simulink model "discrete_control_angle_from_acc"  (Simulink 7.4)
settings: Solver=ode45  StartTime=0.0  StopTime=30.0  RelTol=1e-3
values from neighbouring files (symbols this model uses):
  phi0 = 0.15    [discrete_control_angle_from_acc_Driver.m]    (also in discrete_control_sfunc_Driver.m)
  r_psi0 = 0.1    [discrete_control_angle_from_acc_Driver.m]    (also in discrete_control_sfunc_Driver.m)
  theta0 = 0.15    [discrete_control_angle_from_acc_Driver.m]    (also in discrete_control_sfunc_Driver.m)
undefined symbols (not defined in the file or in its folder): boom, DiscIntNeverNeededParam, f1, f2, f3, f4, f5, g, I_x, I_y, I_z, Ts
libraries: Copter_Library x5
settings Model: Creator=Robert  LastModifiedBy=roczit00

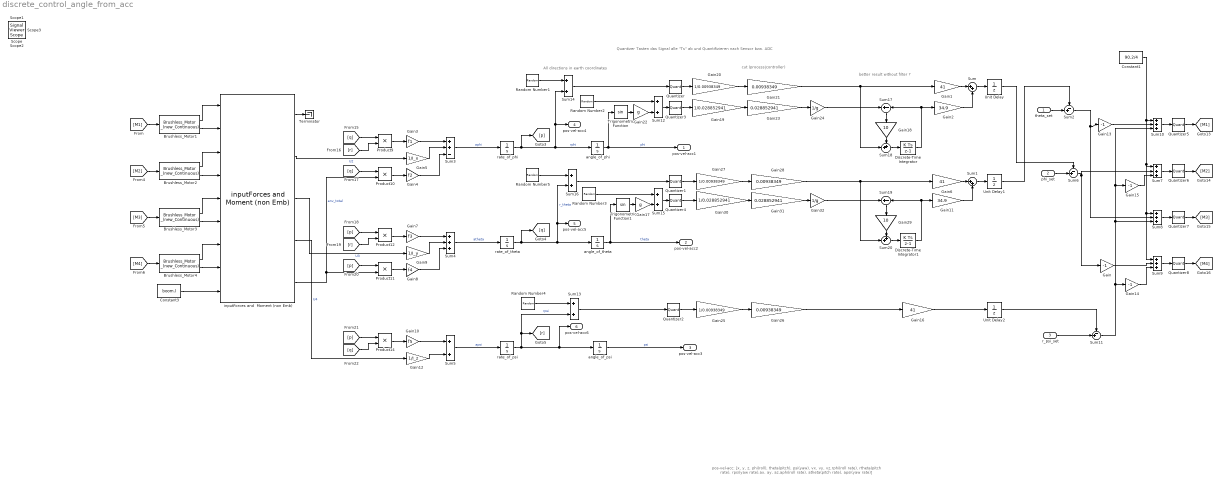
== system discrete_control_angle_from_acc ==
  note: pos-vel-acc: [x, y, z, phi(roll), theta(pitch), psi(yaw), vx, vy, vz,rphi(roll rate), rtheta(pitch rate), rpsi(yaw rate),ax, ay, az,aphi(roll rate), atheta(pitch rate), apsi(yaw rate)]
  note: All directions in earth coordinates
  note: cut (process|controller)
  note: Quantizer Tasten das Signal alle "Ts" ab und Quantifizieren nach Sensor bzw. ADC
  note: better result without filter ?
  theta_set : Inport  OutDataType=fixdt(1, 16)  OutScaling=2^0
  phi_set : Inport  Port=2  OutDataType=fixdt(1, 16)  OutScaling=2^0
  r_psi_set : Inport  Port=3  OutDataType=fixdt(1, 16)  OutScaling=2^0
  Brushless_Motor{1..4} (4 alike) : Copter_Library/Brushless_Motor _(new_Continuous)  SystemSampleTime=-1  M_error=1
  Constant1 : Constant  Value=90.2/4  OutDataType=fixdt(1, 16)  OutScaling=2^0
  Constant3 : Constant  Value=boom.l  OutDataType=fixdt(1, 16)  OutScaling=2^0
  Discrete-Time Integrator : DiscreteIntegrator  InitialCondition=phi0  SampleTime=Ts  OutDataType=fixdt(1, 16)  OutScaling=2^0  ICPrevOutput=DiscIntNeverNeededParam  ICPrevScaledInput=DiscIntNeverNeededParam
  Discrete-Time Integrator1 : DiscreteIntegrator  InitialCondition=theta0  SampleTime=Ts  OutDataType=fixdt(1, 16)  OutScaling=2^0  ICPrevOutput=DiscIntNeverNeededParam  ICPrevScaledInput=DiscIntNeverNeededParam
  Gain{,13..15} (4 alike) : Gain  Gain=-1  ParameterDataType=fixdt(1, 16)  ParameterScaling=2^0  OutDataType=fixdt(1, 16)  OutScaling=2^0
  Gain1 : Gain  Gain=41  ParameterDataType=fixdt(1, 16)  ParameterScaling=2^0  OutDataType=fixdt(1, 16)  OutScaling=2^0
  Gain10 : Gain  Gain=f5  ParameterDataType=fixdt(1, 16)  ParameterScaling=2^0  OutDataType=fixdt(1, 16)  OutScaling=2^0
  Gain11 : Gain  Gain=34.9  ParameterDataType=fixdt(1, 16)  ParameterScaling=2^0  OutDataType=fixdt(1, 16)  OutScaling=2^0
  Gain12 : Gain  Gain=1/I_z  ParameterDataType=fixdt(1, 16)  ParameterScaling=2^0  OutDataType=fixdt(1, 16)  OutScaling=2^0
  Gain16 : Gain  Gain=41  ParameterDataType=fixdt(1, 16)  ParameterScaling=2^0  OutDataType=fixdt(1, 16)  OutScaling=2^0
  Gain17 : Gain  Gain=g  ParameterDataType=fixdt(1, 16)  ParameterScaling=2^0  OutDataType=fixdt(1, 16)  OutScaling=2^0
  Gain18 : Gain  Gain=10  ParameterDataType=fixdt(1, 16)  ParameterScaling=2^0  OutDataType=fixdt(1, 16)  OutScaling=2^0
  Gain19 : Gain  Gain=1/0.028852941  ParameterDataType=fixdt(1, 16)  ParameterScaling=2^0  OutDataType=fixdt(1, 16)  OutScaling=2^0
  Gain2 : Gain  Gain=34.9  ParameterDataType=fixdt(1, 16)  ParameterScaling=2^0  OutDataType=fixdt(1, 16)  OutScaling=2^0
  Gain20 : Gain  Gain=1/0.00938349  ParameterDataType=fixdt(1, 16)  ParameterScaling=2^0  OutDataType=fixdt(1, 16)  OutScaling=2^0
  Gain21 : Gain  Gain=0.00938349  ParameterDataType=fixdt(1, 16)  ParameterScaling=2^0  OutDataType=fixdt(1, 16)  OutScaling=2^0
  Gain22 : Gain  Gain=g  ParameterDataType=fixdt(1, 16)  ParameterScaling=2^0  OutDataType=fixdt(1, 16)  OutScaling=2^0
  Gain23 : Gain  Gain=0.028852941  ParameterDataType=fixdt(1, 16)  ParameterScaling=2^0  OutDataType=fixdt(1, 16)  OutScaling=2^0
  Gain24 : Gain  Gain=1/g  ParameterDataType=fixdt(1, 16)  ParameterScaling=2^0  OutDataType=fixdt(1, 16)  OutScaling=2^0
  Gain25 : Gain  Gain=1/0.00938349  ParameterDataType=fixdt(1, 16)  ParameterScaling=2^0  OutDataType=fixdt(1, 16)  OutScaling=2^0
  Gain26 : Gain  Gain=0.00938349  ParameterDataType=fixdt(1, 16)  ParameterScaling=2^0  OutDataType=fixdt(1, 16)  OutScaling=2^0
  Gain27 : Gain  Gain=1/0.00938349  ParameterDataType=fixdt(1, 16)  ParameterScaling=2^0  OutDataType=fixdt(1, 16)  OutScaling=2^0
  Gain28 : Gain  Gain=0.00938349  ParameterDataType=fixdt(1, 16)  ParameterScaling=2^0  OutDataType=fixdt(1, 16)  OutScaling=2^0
  Gain29 : Gain  Gain=10  ParameterDataType=fixdt(1, 16)  ParameterScaling=2^0  OutDataType=fixdt(1, 16)  OutScaling=2^0
  Gain3 : Gain  Gain=f1  ParameterDataType=fixdt(1, 16)  ParameterScaling=2^0  OutDataType=fixdt(1, 16)  OutScaling=2^0
  Gain30 : Gain  Gain=1/0.028852941  ParameterDataType=fixdt(1, 16)  ParameterScaling=2^0  OutDataType=fixdt(1, 16)  OutScaling=2^0
  Gain31 : Gain  Gain=0.028852941  ParameterDataType=fixdt(1, 16)  ParameterScaling=2^0  OutDataType=fixdt(1, 16)  OutScaling=2^0
  Gain32 : Gain  Gain=1/g  ParameterDataType=fixdt(1, 16)  ParameterScaling=2^0  OutDataType=fixdt(1, 16)  OutScaling=2^0
  Gain4 : Gain  Gain=f2  ParameterDataType=fixdt(1, 16)  ParameterScaling=2^0  OutDataType=fixdt(1, 16)  OutScaling=2^0
  Gain5 : Gain  Gain=1/I_x  ParameterDataType=fixdt(1, 16)  ParameterScaling=2^0  OutDataType=fixdt(1, 16)  OutScaling=2^0
  Gain6 : Gain  Gain=41  ParameterDataType=fixdt(1, 16)  ParameterScaling=2^0  OutDataType=fixdt(1, 16)  OutScaling=2^0
  Gain7 : Gain  Gain=f3  ParameterDataType=fixdt(1, 16)  ParameterScaling=2^0  OutDataType=fixdt(1, 16)  OutScaling=2^0
  Gain8 : Gain  Gain=f4  ParameterDataType=fixdt(1, 16)  ParameterScaling=2^0  OutDataType=fixdt(1, 16)  OutScaling=2^0
  Gain9 : Gain  Gain=1/I_y  ParameterDataType=fixdt(1, 16)  ParameterScaling=2^0  OutDataType=fixdt(1, 16)  OutScaling=2^0
  Product{9..12,14} (5 alike) : Product  OutDataType=fixdt(1, 16)  OutScaling=2^0  RndMeth=Zero
  Quantizer : Quantizer  QuantizationInterval=0.00938349  SampleTime=Ts
  Quantizer1 : Quantizer  QuantizationInterval=0.00938349  SampleTime=Ts
  Quantizer2 : Quantizer  QuantizationInterval=0.00938349  SampleTime=Ts
  Quantizer3 : Quantizer  QuantizationInterval=0.028852941  SampleTime=Ts
  Quantizer4 : Quantizer  QuantizationInterval=0.003  SampleTime=Ts
  Quantizer{5..8} (4 alike) : Quantizer  QuantizationInterval=1  SampleTime=Ts
  Random Number1 : RandomNumber  Variance=3.0462e-8  Seed=45632  SampleTime=0.01
  Random Number2 : RandomNumber  Variance=0.0003  Seed=4564  SampleTime=0.01
  Random Number3 : RandomNumber  Variance=0.0003  Seed=676  SampleTime=Ts
  Random Number4 : RandomNumber  Variance=3.0462e-8  Seed=1634  SampleTime=0.01
  Random Number5 : RandomNumber  Variance=3.0462e-8  Seed=4731  SampleTime=0.01
  Sum : Sum  Inputs=|++  OutDataType=fixdt(1, 16)  OutScaling=2^0
  Sum1 : Sum  Inputs=|++  OutDataType=fixdt(1, 16)  OutScaling=2^0
  Sum{4,7..10} (5 alike) : Sum  Inputs=+++  OutDataType=fixdt(1, 16)  OutScaling=2^0
  Sum11 : Sum  Inputs=-+|  OutDataType=fixdt(1, 16)  OutScaling=2^0
  Sum{5,12..16} (6 alike) : Sum  OutDataType=fixdt(1, 16)  OutScaling=2^0
  Sum17 : Sum  Inputs=+|-  OutDataType=fixdt(1, 16)  OutScaling=2^0
  Sum18 : Sum  Inputs=++|  OutDataType=fixdt(1, 16)  OutScaling=2^0
  Sum19 : Sum  Inputs=+|-  OutDataType=fixdt(1, 16)  OutScaling=2^0
  Sum2 : Sum  Inputs=-+|  OutDataType=fixdt(1, 16)  OutScaling=2^0
  Sum20 : Sum  Inputs=++|  OutDataType=fixdt(1, 16)  OutScaling=2^0
  Sum3 : Sum  Inputs=++-  OutDataType=fixdt(1, 16)  OutScaling=2^0
  Sum6 : Sum  Inputs=-+|  OutDataType=fixdt(1, 16)  OutScaling=2^0
  Terminator : Terminator
  Trigonometric Function : Trigonometry
  Trigonometric Function1 : Trigonometry
  Unit Delay : UnitDelay  SampleTime=Ts
  Unit Delay1 : UnitDelay  SampleTime=Ts
  Unit Delay2 : UnitDelay  SampleTime=Ts
  angle_of_phi : Integrator  InitialCondition=phi0
  angle_of_psi : Integrator
  angle_of_theta : Integrator  InitialCondition=theta0
  inputForces and  Moment (non Emb) : Copter_Library/inputForces and  Moment (non Emb)  SystemSampleTime=-1
  rate_of_phi : Integrator
  rate_of_psi : Integrator  InitialCondition=r_psi0
  rate_of_theta : Integrator
  pos-vel-acc1 : Outport  OutDataType=fixdt(1, 16)  OutScaling=2^0
  pos-vel-acc2 : Outport  Port=2  OutDataType=fixdt(1, 16)  OutScaling=2^0
  pos-vel-acc3 : Outport  Port=3  OutDataType=fixdt(1, 16)  OutScaling=2^0
  pos-vel-acc4 : Outport  Port=4  OutDataType=fixdt(1, 16)  OutScaling=2^0
  pos-vel-acc5 : Outport  Port=5  OutDataType=fixdt(1, 16)  OutScaling=2^0
  pos-vel-acc6 : Outport  Port=6  OutDataType=fixdt(1, 16)  OutScaling=2^0
  Scope : SignalViewerScope  IOType=viewer  ZoomMode=yonly  LegendLocations="235.3333           183            72      20.33333"  RefreshTime=0.035000
      settings: ShowLegends=on
  Scope1 : SignalViewerScope  IOType=viewer  ZoomMode=yonly  LegendLocations="225.3333           183            82      20.33333"  RefreshTime=0.035000
      settings: ShowLegends=on
  Scope2 : SignalViewerScope  IOType=viewer  ZoomMode=yonly  LegendLocations="220.3333           183            74      20.33333"  RefreshTime=0.035000
      settings: ShowLegends=on  SaveName=ScopeData2
  Scope3 : SignalViewerScope  IOType=viewer  ZoomMode=xonly  RefreshTime=0.035000
      settings: ShowLegends=on  SaveName=ScopeData3
  wires:
  Constant3/1 -> inputForces and  Moment (non Emb)/9
  Sum5/1 -> rate_of_psi/1  "apsi"
  inputForces and  Moment (non Emb)/4 -> Gain12/1  "U4"
  Gain12/1 -> Sum5/2
  Gain10/1 -> Sum5/1
  Product14/1 -> Gain10/1
  [q] -> Product14/2
  [p] -> Product14/1
  Sum4/1 -> rate_of_theta/1  "atheta"
  inputForces and  Moment (non Emb)/3 -> Gain9/1  "U3"
  Gain8/1 -> Sum4/3
  Gain9/1 -> Sum4/2
  Product11/1 -> Gain8/1
  [p] -> Product11/1
  Gain7/1 -> Sum4/1
  Product12/1 -> Gain7/1
  [r] -> Product12/2
  [p] -> Product12/1
  Sum3/1 -> rate_of_phi/1  "aphi"
  Gain4/1 -> Sum3/3
  Gain5/1 -> Sum3/2
  inputForces and  Moment (non Emb)/2 -> Gain5/1  "U2"
  Product10/1 -> Gain4/1
  [q] -> Product10/1
  Gain3/1 -> Sum3/1
  Product9/1 -> Gain3/1
  [r] -> Product9/2
  [q] -> Product9/1
  inputForces and  Moment (non Emb)/5 -> Product11/2, Product10/2  "anv_total"
  angle_of_phi/1 -> pos-vel-acc1/1, Trigonometric Function/1  "phi"
  angle_of_theta/1 -> pos-vel-acc2/1, Trigonometric Function1/1  "theta"
  angle_of_psi/1 -> pos-vel-acc3/1  "psi"
  rate_of_phi/1 -> [p], angle_of_phi/1, pos-vel-acc4/1, Sum14/2  "rphi"
  rate_of_theta/1 -> angle_of_theta/1, pos-vel-acc5/1, Sum16/2, [q]  "r_theta"
  rate_of_psi/1 -> angle_of_psi/1, pos-vel-acc6/1, [r], Sum13/2  "rpsi"
  Brushless_Motor1/1 -> inputForces and  Moment (non Emb)/1
  Brushless_Motor1/2 -> inputForces and  Moment (non Emb)/2
  Brushless_Motor2/1 -> inputForces and  Moment (non Emb)/3
  Brushless_Motor2/2 -> inputForces and  Moment (non Emb)/4
  Brushless_Motor3/1 -> inputForces and  Moment (non Emb)/5
  Brushless_Motor3/2 -> inputForces and  Moment (non Emb)/6
  Brushless_Motor4/1 -> inputForces and  Moment (non Emb)/7
  Brushless_Motor4/2 -> inputForces and  Moment (non Emb)/8
  Gain1/1 -> Sum/1
  Gain2/1 -> Sum/2
  Gain6/1 -> Sum1/1
  Gain11/1 -> Sum1/2
  inputForces and  Moment (non Emb)/1 -> Terminator/1
  Sum/1 -> Unit Delay/1
  Sum1/1 -> Unit Delay1/1
  Gain16/1 -> Unit Delay2/1
  Random Number2/1 -> Sum12/1
  Random Number1/1 -> Sum14/1
  Random Number3/1 -> Sum15/1
  Random Number5/1 -> Sum16/1
  Random Number4/1 -> Sum13/1
  Sum14/1 -> Quantizer/1
  Sum16/1 -> Quantizer1/1
  Sum13/1 -> Quantizer2/1
  Sum12/1 -> Quantizer3/1
  Sum15/1 -> Quantizer4/1
  Unit Delay2/1 -> Sum11/1
  Unit Delay1/1 -> Sum2/1
  Unit Delay/1 -> Sum6/1
  [M1] -> Brushless_Motor1/1
  theta_set/1 -> Sum2/2
  Sum2/1 -> Gain13/1, Sum8/2
  phi_set/1 -> Sum6/2
  Sum6/1 -> Gain/1, Sum7/2
  Constant1/1 -> Sum10/1, Sum7/1, Sum8/1, Sum9/1
  Gain13/1 -> Sum10/2
  Gain/1 -> Sum9/2
  r_psi_set/1 -> Sum11/2
  Gain15/1 -> Sum7/3
  Sum11/1 -> Gain14/1, Sum8/3, Gain15/1, Sum10/3
  Gain14/1 -> Sum9/3
  Sum10/1 -> Quantizer5/1
  Sum7/1 -> Quantizer6/1
  Sum8/1 -> Quantizer7/1
  Sum9/1 -> Quantizer8/1
  [M2] -> Brushless_Motor2/1
  [M3] -> Brushless_Motor3/1
  [M4] -> Brushless_Motor4/1
  Quantizer5/1 -> [M1]
  Quantizer6/1 -> [M2]
  Quantizer7/1 -> [M3]
  Quantizer8/1 -> [M4]
  Sum18/1 -> Discrete-Time Integrator/1
  Gain18/1 -> Sum18/1
  Sum17/1 -> Gain18/1
  Quantizer/1 -> Gain20/1
  Gain20/1 -> Gain21/1
  Trigonometric Function/1 -> Gain22/1
  Gain22/1 -> Sum12/2
  Trigonometric Function1/1 -> Gain17/1
  Gain17/1 -> Sum15/2
  Gain21/1 -> Sum18/2, Gain1/1
  Gain19/1 -> Gain23/1
  Quantizer3/1 -> Gain19/1
  Gain23/1 -> Gain24/1
  Gain24/1 -> Sum17/1
  Gain25/1 -> Gain26/1
  Gain27/1 -> Gain28/1
  Quantizer1/1 -> Gain27/1
  Gain28/1 -> Gain6/1, Sum20/2
  Quantizer2/1 -> Gain25/1
  Gain26/1 -> Gain16/1
  Sum20/1 -> Discrete-Time Integrator1/1
  Gain29/1 -> Sum20/1
  Sum19/1 -> Gain29/1
  Gain30/1 -> Gain31/1
  Gain31/1 -> Gain32/1
  Gain32/1 -> Sum19/1
  Quantizer4/1 -> Gain30/1
  Discrete-Time Integrator/1 -> Gain2/1, Sum17/2
  Discrete-Time Integrator1/1 -> Gain11/1, Sum19/2
